simulink model "CorWf_TestBed"  (R2012b)
settings: Solver=FixedStepDiscrete  StartTime=0.0  StopTime=1  FixedStep=1  RelTol=1e-3
undefined symbols (not defined in the file): MWS
libraries: Lib_Cntrl_CorrectedFuelFlow_TMATS x1
settings Model: Creator=jwchapm2  LastModifiedBy=jwchapm2

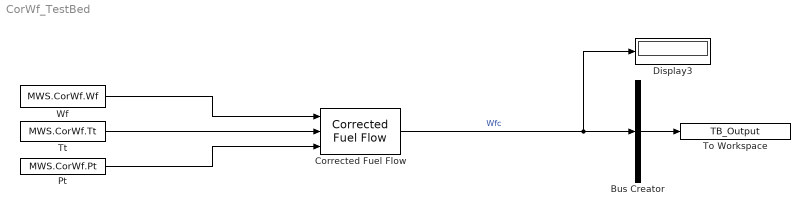
== system CorWf_TestBed ==
  Bus Creator : BusCreator  Inputs=1
  Corrected Fuel Flow : Lib_Cntrl_CorrectedFuelFlow_TMATS/Corrected Fuel Flow  C_TSTD_M=MWS.CorWf.TST  C_PSTD_M=MWS.CorWf.PST
  Display3 : Display
  Pt : Constant  Value=MWS.CorWf.Pt
  To Workspace : ToWorkspace  VariableName=TB_Output  SampleTime=-1
  Tt : Constant  Value=MWS.CorWf.Tt
  Wf : Constant  Value=MWS.CorWf.Wf
  wires:
  Wf/1 -> Corrected Fuel Flow/1
  Tt/1 -> Corrected Fuel Flow/2
  Pt/1 -> Corrected Fuel Flow/3
  Corrected Fuel Flow/1 -> Display3/1, Bus Creator/1  "Wfc"
  Bus Creator/1 -> To Workspace/1
